simulink model "model_1"  (R2023a)
settings: Solver=VariableStepAuto  StartTime=0.0  StopTime=10  RelTol=1e-3
values from neighbouring files (symbols this model uses):
  Ac = [-2 -2 -1; 1 0 0; 0 1 0]    [data_1.m]
  Ad1 = expm(Ac*dt1)    [data_1.m]
  Ad2 = expm(Ac*dt2)    [data_1.m]
  Ad3 = expm(Ac*dt3)    [data_1.m]
  Bc = [2; 0; 0]    [data_1.m]
  Bd1 = inv(Ac)*(Ad1 - eye(3,3)) *Bc    [data_1.m]
  Bd2 = inv(Ac)*(Ad2 - eye(3,3)) *Bc    [data_1.m]
  Bd3 = inv(Ac)*(Ad3 - eye(3,3)) *Bc    [data_1.m]
  Cc = [-0.5 -0.5 -0.5]    [data_1.m]
  Cd1 = Cc    [data_1.m]
  Cd2 = Cc    [data_1.m]
  Cd3 = Cc    [data_1.m]
  Dc = [1]    [data_1.m]
  Dd1 = Dc    [data_1.m]
  Dd2 = Dc    [data_1.m]
  Dd3 = Dc    [data_1.m]
  dt1 = 0.2    [data_1.m]
  dt2 = 1/30    (= 0.0333333333333)    [data_1.m]
  dt3 = 0.01    [data_1.m]
  W = tf([1 1 1 0],[1 2 2 1])    [data_1.m]
settings Model: Creator=TheMix  LastModifiedBy=TheMix

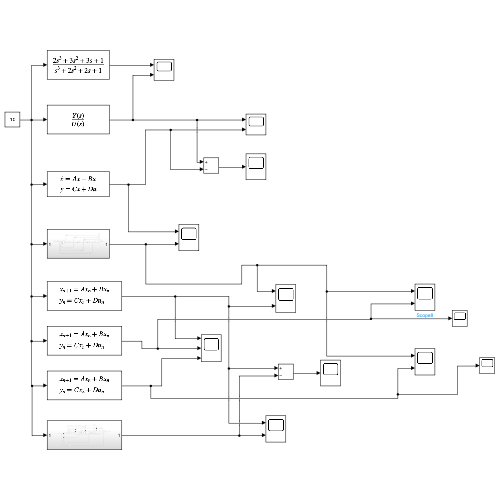
[thumbnail: Simulink's stored preview of the top-level diagram]
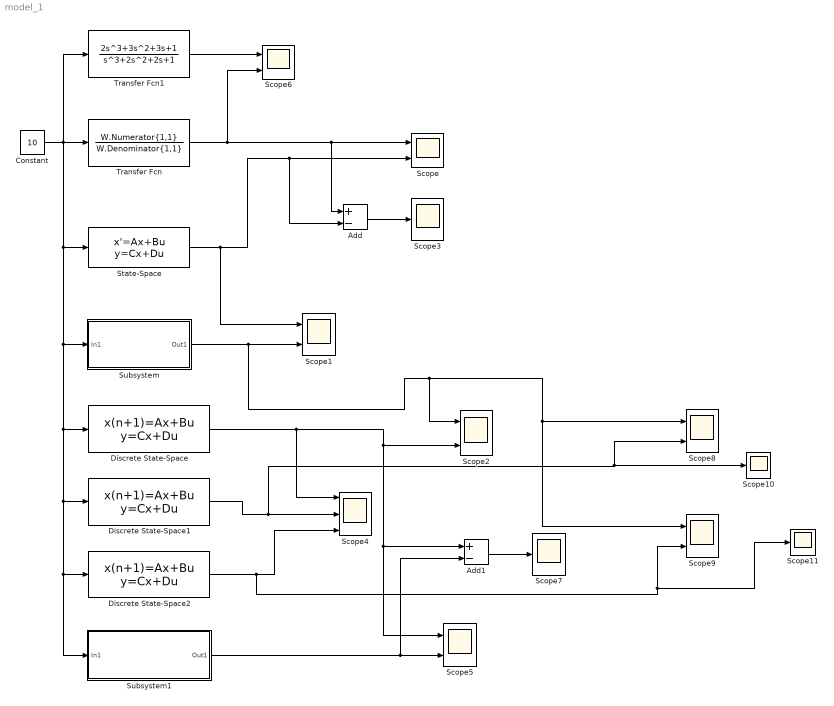
== system model_1 ==
  Add : Sum  Inputs=+-
  Add1 : Sum  Inputs=+-
  Constant : Constant  Value=10
  Discrete State-Space : DiscreteStateSpace  A=Ad1  B=Bd1  C=Cd1  D=Dd1  SampleTime=dt1
  Discrete State-Space1 : DiscreteStateSpace  A=Ad2  B=Bd2  C=Cd2  D=Dd2  SampleTime=dt2
  Discrete State-Space2 : DiscreteStateSpace  A=Ad3  B=Bd3  C=Cd3  D=Dd3  SampleTime=dt3
  Scope{,1..2,5..6,8..9} (7 alike) : Scope  NumInputPorts=2
  Scope{3,7,10..11} (4 alike) : Scope
  Scope4 : Scope  NumInputPorts=3
  State-Space : StateSpace  A=Ac  B=Bc  C=Cc  D=Dc  InitialCondition=0
  Subsystem : Subsystem
  Subsystem1 : Subsystem
  Transfer Fcn : TransferFcn  Numerator=W.Numerator{1,1}  Denominator=W.Denominator{1,1}
  Transfer Fcn1 : TransferFcn  Numerator=[2 3 3 1]  Denominator=[1 2 2 1]
  wires:
  Transfer Fcn/1 -> Scope6/2, Add/1, Scope/1
  Constant/1 -> Transfer Fcn1/1, Subsystem1/1(In1), Discrete State-Space2/1, Discrete State-Space1/1, Discrete State-Space/1, Subsystem/1(In1), State-Space/1, Transfer Fcn/1
  Add/1 -> Scope3/1
  State-Space/1 -> Scope1/1, Add/2, Scope/2
  Subsystem/1(Out1) -> Scope2/1, Scope9/1, Scope8/1, Scope1/2
  Discrete State-Space/1 -> Scope4/1, Scope2/2, Add1/1, Scope5/1
  Discrete State-Space1/1 -> Scope8/2, Scope10/1, Scope4/2
  Discrete State-Space2/1 -> Scope11/1, Scope9/2, Scope4/3
  Subsystem1/1(Out1) -> Add1/2, Scope5/2
  Transfer Fcn1/1 -> Scope6/1
  Add1/1 -> Scope7/1

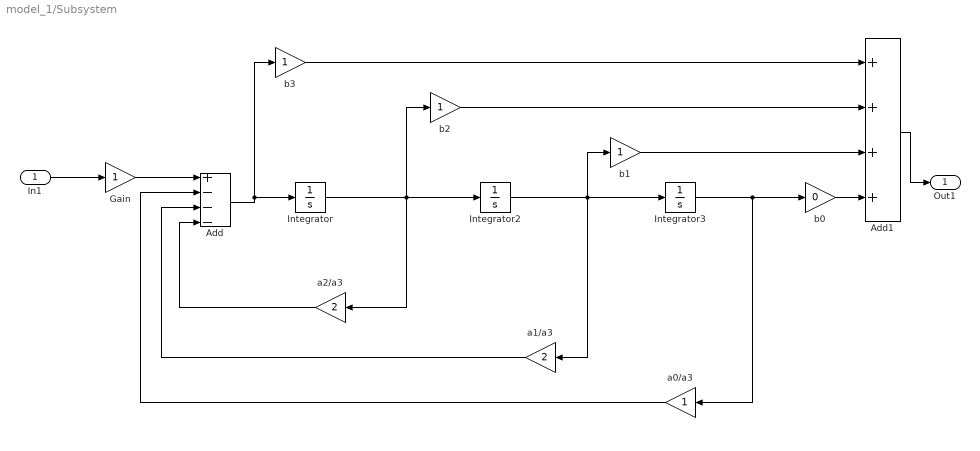
== system model_1/Subsystem ==
  In1 : Inport
  Add : Sum  Inputs=+---
  Add1 : Sum  Inputs=++++
  Gain : Gain
  Integrator : Integrator
  Integrator2 : Integrator
  Integrator3 : Integrator
  a0/a3 : Gain
  a1/a3 : Gain  Gain=2
  a2/a3 : Gain  Gain=2
  b0 : Gain  Gain=0
  b1 : Gain
  b2 : Gain
  b3 : Gain
  Out1 : Outport
  wires:
  In1/1 -> Gain/1
  Gain/1 -> Add/1
  Add/1 -> b3/1, Integrator/1
  Add1/1 -> Out1/1
  b0/1 -> Add1/4
  Integrator3/1 -> a0/a3/1, b0/1
  Integrator2/1 -> b1/1, a1/a3/1, Integrator3/1
  Integrator/1 -> a2/a3/1, b2/1, Integrator2/1
  a2/a3/1 -> Add/4
  a1/a3/1 -> Add/3
  a0/a3/1 -> Add/2
  b1/1 -> Add1/3
  b2/1 -> Add1/2
  b3/1 -> Add1/1

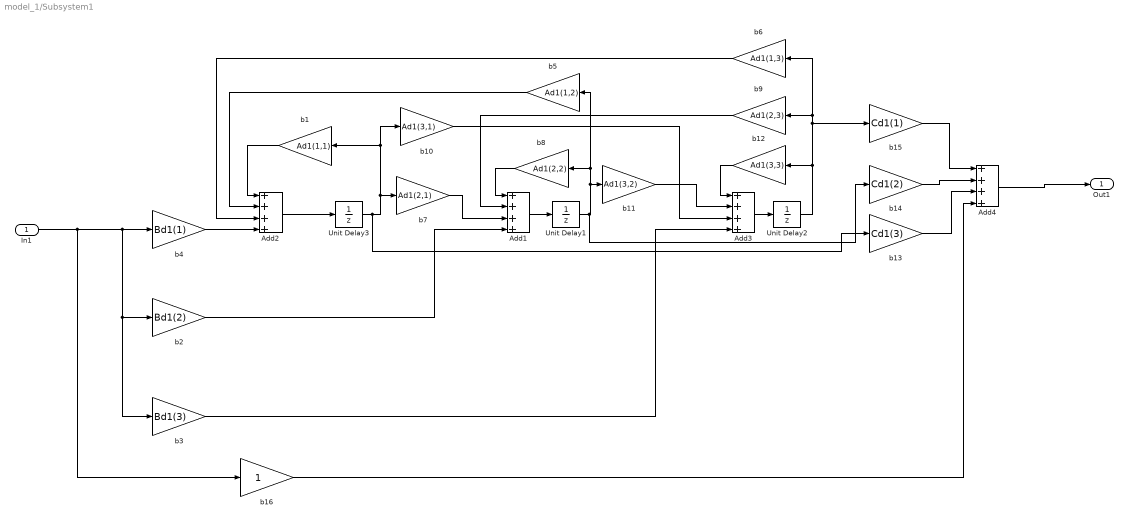
== system model_1/Subsystem1 ==
  In1 : Inport
  Add{1..4} (4 alike) : Sum  Inputs=++++
  Unit Delay1 : UnitDelay  SampleTime=-1  HasFrameUpgradeWarning=on
  Unit Delay2 : UnitDelay  SampleTime=-1  HasFrameUpgradeWarning=on
  Unit Delay3 : UnitDelay  SampleTime=-1  HasFrameUpgradeWarning=on
  b1 : Gain  Gain=Ad1(1,1)
  b10 : Gain  Gain=Ad1(3,1)
  b11 : Gain  Gain=Ad1(3,2)
  b12 : Gain  Gain=Ad1(3,3)
  b13 : Gain  Gain=Cd1(3)
  b14 : Gain  Gain=Cd1(2)
  b15 : Gain  Gain=Cd1(1)
  b16 : Gain
  b2 : Gain  Gain=Bd1(2)
  b3 : Gain  Gain=Bd1(3)
  b4 : Gain  Gain=Bd1(1)
  b5 : Gain  Gain=Ad1(1,2)
  b6 : Gain  Gain=Ad1(1,3)
  b7 : Gain  Gain=Ad1(2,1)
  b8 : Gain  Gain=Ad1(2,2)
  b9 : Gain  Gain=Ad1(2,3)
  Out1 : Outport
  wires:
  b4/1 -> Add2/4
  Add2/1 -> Unit Delay3/1
  Unit Delay3/1 -> b13/1, b10/1, b1/1, b7/1
  b1/1 -> Add2/1
  Unit Delay1/1 -> b14/1, b11/1, b5/1, b8/1
  b5/1 -> Add2/2
  Unit Delay2/1 -> b12/1, b15/1, b6/1, b9/1
  b6/1 -> Add2/3
  b2/1 -> Add1/4
  Add1/1 -> Unit Delay1/1
  Add3/1 -> Unit Delay2/1
  b3/1 -> Add3/4
  b7/1 -> Add1/3
  b8/1 -> Add1/1
  b9/1 -> Add1/2
  b10/1 -> Add3/3
  b11/1 -> Add3/2
  b12/1 -> Add3/1
  b13/1 -> Add4/3
  b14/1 -> Add4/2
  b15/1 -> Add4/1
  Add4/1 -> Out1/1
  In1/1 -> b16/1, b2/1, b3/1, b4/1
  b16/1 -> Add4/4
